simulink model "AUDI"  (R2019b)
settings: Solver=VariableStepAuto  StartTime=0.0  StopTime=100  RelTol=1e-3  AbsTol=1e-3  EnableMultiTasking=on
model workspace (MATLAB code in the model file):
  | v0                 = 15; % Initial vehicle speed
  | wheel_radius = 0.3; % Wheel radius
  | k                   = 1e-2; % Motor losses (W/(N*M)^2)
  | t_torque        = 0.02; % Electric motor time constant
  | gear_ratio     = 4.27;
values from neighbouring files (symbols this model uses):
  dc_battery_internal_resistance = 1e-6    (= 1e-06)    [audi_a3_parameters.m]
  gravitational_acceleration = 9.81    [audi_a3_parameters.m]
  Ki = 60    [audi_a3_parameters.m]
  Kp = 60    [audi_a3_parameters.m]
  speed_controller_lower_limit = -400    [audi_a3_parameters.m]
  speed_controller_upper_limit = 400    [audi_a3_parameters.m]
libraries: fl_lib x36, nesl_utility x11, sdl_lib x5
CloseFcn:
  | try,close(h1_sdl_hybrid_parallel),end
  | clear h1_sdl_hybrid_parallel
  | try,close(h2_sdl_hybrid_parallel),end
  | clear h2_sdl_hybrid_parallel
  | 
  | 
  | clear simlog_sdl_hybrid_parallel
Description:
  | Parallel Hybrid Transmission
settings Model: FPTRunName=Active  Creator=MathWorks  LastModifiedBy=Matheus Elyasha
settings SolverCC: AutoScaleAbsTol=off
settings DataIOCC: LimitDataPoints=on  MaxDataPoints=10000  SaveFormat=Array  SignalLoggingSaveFormat=ModelDataLogs  ReturnWorkspaceOutputs=off  SignalLoggingName=logsout_sdl_hybrid_parallel
settings OptimizationCC: ExpressionDepthLimit=2147483647  LifeSpan=inf
settings DebuggingCC: StateNameClashWarn=warning  PregeneratedLibrarySubsystemCodeDiagnostic=none  SFUnexpectedBacktrackingDiag=warning  SFNoUnconditionalDefaultTransitionDiag=warning  SFExecutionAtInitializationDiag=none  ArithmeticOperatorsInVariantConditions=warning
settings HardwareCC: ProdBitPerPointer=32  ProdBitPerSizeT=32  ProdBitPerPtrDiffT=32  ProdLargestAtomicFloat=None  ProdIntDivRoundTo=Undefined  ProdEndianess=Unspecified  ProdWordSize=32  ProdHWDeviceType=32-bit Generic
settings ModelReferenceCC: PropagateSignalLabelsOutOfModel=off
settings SFSimCC: SimUseLocalCustomCode=off  CustomCodeUndefinedFunction=UseInterfaceOnly
settings RTWCC: RTWUseLocalCustomCode=off
settings CodeAppCC: StateflowObjectComments=on
settings GRTTargetCC: TargetLangStandard=C89/C90 (ANSI)  GeneratePreprocessorConditionals=Disable all  CombineOutputUpdateFcns=off  GRTInterface=on
settings ConfigComp: CovMetricSettings=dw  CovHtmlReporting=on  CovSaveCumulativeToWorkspaceVar=on  CovSaveSingleToWorkspaceVar=on  CovShowResultsExplorer=off  CovExternalEMLEnable=off
settings SimscapeCC: SimscapeLogType=all  SimscapeLogSimulationStatistics=on  SimscapeLogName=simlog_sdl_hybrid_parallel  SimscapeLogDataHistory=10000

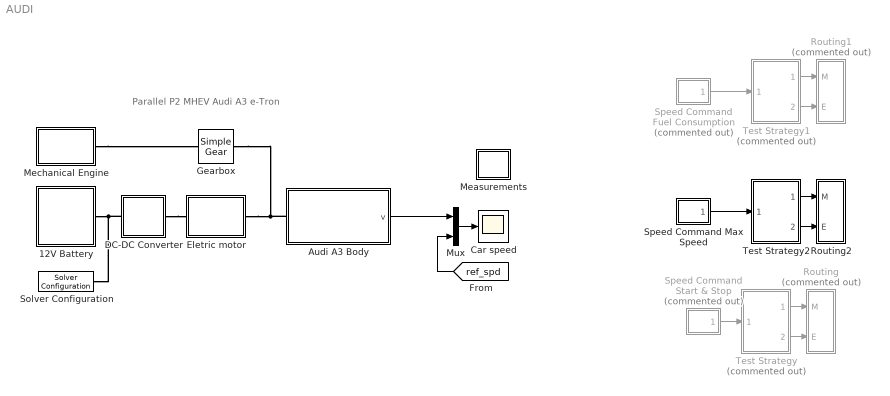
== system AUDI ==
  note: Parallel P2 MHEV Audi A3 e-Tron
  12V Battery : Subsystem
      mask Display:
      | % Plot points to set plot range
      | color('white');plot(1.5, 2.5);plot(-1.5, -2)
      | color('black');
      | % Battery icon
      | plot([0 0], [2.5 1.3])
      | plot([0 0], [-0.6 -1.6])
      | patch([-1 1 1 -1]*0.4, [1 1 -1 -1]*0.15+0.7,[0;0;0]);
      | patch([-1 1 1 -1]*0.4, [1 1 -1 -1]*0.15-0.6,[0;0;0]);
      | patch([-1 1 1 -1]*0.8, [1 1 -1 -1]*0.15+1.3,[0;0;0]);
      | patch([-1 1 1 -1]*0.8, [1 1 -1 -1]*0.15+0.0,[0;0;0]);
  Audi A3 Body : Subsystem
      mask Display:
      | color('white')
      | plot(-120,-60); plot(120,50);
      | color('black')
      | plot(sin(0:0.1:6*pi)*15-70,cos(0:0.1:6*pi)*15-30);
      | plot(sin(0:0.1:6*pi)*15+70,cos(0:0.1:6*pi)*15-30);
      | plot([-88 -95 -99 -99 -95 -75 -65 -50 -46 10 30 34 80 85 90 93 95 93 90 88],[-30 -28 -23 -5 0 5 10 20 21 21 0 -2 -7 -9 -13 -17 -25 -28 -30 -30])
      | plot([-88 -95 -99 -99 -95 -75 -65 -50 -46 10 30 34 80 85 90 93 95 93 90 88],[-30 -28 -23 -5 0 5 10 20 21 21 0 -2 -7 -9 -13 -17 -25 -28 -30 -30]-1)
      | plot([-88 -95 -99 -99 -95 -75 -65 -50 -46 10 30 34 80 85 90 93 95 93 90 88]+1,[-30 -28 -23 -5 0 5 10 20 21 21 0 -2 -7 -9 -13 -17 -25 -28 -30 -30])
      | plot([-50 50],[-30 -30])
  Car speed : Scope
  DC-DC Converter : Subsystem
      mask Display:
      | patch([-0.9 -1 -1 0.9 1 1 -0.9],[-1 -1 -0.9 1 1 0.9 -1],[0 0 0])
      | 
      | patch([-0.8 -0.1 -0.1 -0.8],[0.85 0.85 0.75 0.75],[0 0 0])
      | patch([-0.8 -0.55 -0.55 -0.8],[0.65 0.65 0.55 0.55],[0 0 0])
      | patch([-0.35 -0.1 -0.1 -0.35],[0.65 0.65 0.55 0.55],[0 0 0])
      | 
      | patch([-0.8 -0.1 -0.1 -0.8]*-1,[0.65 0.65 0.55 0.55]*-1,[0 0 0])
      | patch([-0.8 -0.55 -0.55 -0.8]*-1,[0.85 0.85 0.75 0.75]*-1,[0 0 0])
      | patch([-0.35 -0.1 -0.1 -0.35]*-1,[0.85 0.85 0.75 0.75]*-1,[0 0 0])
  Eletric motor : Subsystem
      mask Display:
      | % Circle
      | plot(sin(0:0.1:2.2*pi)*0.9,cos(0:0.1:2.2*pi)*0.9);
      | 
      | % In/out
      | plot([-1.1 -0.9],[0 0]);
      | plot([1.1 0.9],[0 0]);
      | 
      | % 'M'
      | plot([0.5 0.5],[-0.5 0.5]);
      | plot([-0.5 -0.5],[-0.5 0.5]);
      | plot([0.5 0],[0.5 -0.5]);
      | plot([-0.5 0],[0.5 -0.5]);
      | 
      | % Plot points to set plot range
      | color('white');plot(1.9,1.2);plot(-1.9,-1.2)
      | color('black');
  Gearbox : sdl_lib/Gears/Simple Gear  ratio=gear_ratio  rotation_direction=1  friction_model=sdl.enum.gear_efficiencies_load.constant  T_noload=0.1 N*m  T_nom=5 N*m  efficiency_nom=0.8  efficiency=gearbox_efficiency  mu_visc=gearbox_viscous_friction_coefficient_at_B_and_F N*m/(rad/s)  w_thr=0.01 rad/s  pwr_thr=gearbox_follower_power_threshold W  enable_faults=simscape.enum.onoff.off  efficiency_fault=0.05  external_fault=simscape.enum.onoff.off  temporal_fault=simscape.enum.onoff.off  fault_time=5 s  fault_angles=pi / 12 rad  report_fault=1  temperature_TLU=[ 280 300 320 ] K  load_TLU=[ 1 5 10 ] N*m  efficiency_TLU=[ 0.95 0.9 0.85 ]  efficiency_TLU2=[ 0.85 0.8 0.75; 0.95 0.9 0.85; 0.85 0.8 0.7 ]  thermal_mass=50 J/K  T_init=300 K
      settings: SourceProductName=Simscape Driveline
  Measurements : Subsystem
  Mechanical Engine : Subsystem
      mask Display:
      | patch([0 374 374 0 0],[183 40 40 183 183],[1 1 1]);
      | plot([200.294537656123;201.704177092068;202.879954177142;203.81054553527;204.486989062962;204.902770239264;205.053884864158;204.938877621199;204.558856093007;203.917480094638;203.02092642757;201.877829393721;200.499197642409;198.898308151034;197.090578360535;195.093417696999;192.926059909376;191.349221415216], [79.0962651705123;81.4129472419303;83.856642682368;86.4038173688741;89.0299406167901;91.7097214236537;94.4173520353776;97.1267564890293;99.8118417386092;102.446748945347;105.006102512455;107.465254465996;109.80052182835;111.989414698229;114.010852840726;115.845368701499;117.475294889959;118.468271604945])
      | plot([180.070315486255;177.215173525063;174.340173090774;171.473002009205;168.641272705228;165.872256280019;163.192619875453;160.628169854943;158.203603274058;155.942270034374;153.865948011161;151.994633320535;150.346347745932;148.936965178479;147.780058742747;146.886770080143;146.265702048809;145.922835873396;145.861473542603;146.08220600922;146.58290749893;147.358755982674;148.402279615432;149.703428694174;151.249672441989;153.026119686324;155.015662269112;157.199139807684;159.555524219735;162.062122235246;164.694793945081;167.42818528151;170.23597219174;173.091114152932;175.966114587221;178.83328566879;181.665014972767;184.434031397976;185.486929355725], [123.25590763568;123.598773811093;123.660136141886;123.439403675268;122.938702185559;122.162853701815;121.119330069056;119.818180990315;118.2719372425;116.495489998164;114.505947415377;112.322469876805;109.966085464754;107.459487449243;104.826815739408;102.093424402979;99.2856374927491;96.4304955315569;93.5554950972677;90.688324015699;87.8565947117214;85.0875782865128;82.4079418819464;79.8434918614364;77.4189252805513;75.1575920408679;73.081270017655;71.2099553270291;69.5616697524256;68.1522871849724;66.9953807492411;66.1020920866371;65.4810240553025;65.1381578798894;65.0767955490969;65.2975280157144;65.7982295054238;66.5740779891678;66.9481130562871])
      | plot([182.088349247351;182.056804583223;181.962474383197;181.806267098667;181.589687091173;181.314820144583;180.98431337785;180.601349751811;180.169617415534;179.693274187426;179.176907513169;178.625490286111;178.044332955585;177.439032384376;176.815417947876;176.17949539401;175.537389004603;174.895282615196;174.25936006133;173.63574562483;173.030445053621;172.449287723095;171.897870496037;171.38150382178;170.905160593672;170.473428257395;170.090464631356;169.759957864623;169.485090918033;169.268510910539;169.112303626009;169.017973425983;168.986428761855;169.017973425983;169.112303626009;169.268510910539;169.485090918033;169.759957864623;170.090464631356;170.473428257395;170.905160593672;171.38150382178;171.897870496037;172.449287723095;173.030445053621;173.63574562483;174.25936006133;174.895282615196;175.537389004603;176.17949539401;176.815417947876;177.439032384376;178.044332955585;178.625490286111;179.176907513169;179.693274187426;180.169617415534;180.601349751811;180.98431337785;181.314820144583;181.589687091173;181.806267098667;181.962474383197;182.056804583223;182.088349247351;182.088349247351], [94.3432759959251;93.7073437064164;93.0775357924916;92.4599176486499;91.8604372752408;91.2848679959696;90.7387528576339;90.2273512475527;89.7555882427917;89.3280071789786;88.9487258954975;88.6213970784445;88.3491730832641;88.1346755758426;87.9799702844327;87.8865471055612;87.8553057555109;87.8865471055612;87.9799702844327;88.1346755758426;88.3491730832641;88.6213970784445;88.9487258954975;89.3280071789786;89.7555882427917;90.2273512475527;90.7387528576339;91.2848679959696;91.8604372752408;92.4599176486499;93.0775357924916;93.7073437064164;94.3432759959251;94.9792082854337;95.6090161993586;96.2266343432003;96.8261147166093;97.4016839958805;97.9477991342162;98.4592007442974;98.9309637490584;99.3585448128716;99.7378260963527;100.065154913406;100.337378908586;100.551876416008;100.706581707417;100.800004886289;100.831246236339;100.800004886289;100.706581707417;100.551876416008;100.337378908586;100.065154913406;99.7378260963526;99.3585448128716;98.9309637490584;98.4592007442974;97.9477991342162;97.4016839958805;96.8261147166093;96.2266343432003;95.6090161993586;94.9792082854338;94.3432759959251;94.3432759959251])
      | plot([201.615249970928;201.583705306799;201.489375106774;201.333167822243;201.11658781475;200.84172086816;200.511214101427;200.128250475388;199.69651813911;199.220174911002;198.703808236745;198.152391009688;197.571233679162;196.965933107953;196.342318671452;195.706396117586;195.06428972818;194.422183338773;193.786260784907;193.162646348407;192.557345777197;191.976188446671;191.424771219614;190.908404545357;190.432061317249;190.000328980971;189.617365354932;189.286858588199;189.011991641609;188.795411634116;188.639204349585;188.54487414956;188.513329485431;188.54487414956;188.639204349585;188.795411634116;189.011991641609;189.286858588199;189.617365354932;190.000328980971;190.432061317249;190.908404545357;191.424771219614;191.976188446671;192.557345777197;193.162646348407;193.786260784907;194.422183338773;195.06428972818;195.706396117586;196.342318671452;196.965933107953;197.571233679162;198.152391009688;198.703808236745;199.220174911002;199.69651813911;200.128250475388;200.511214101427;200.84172086816;201.11658781475;201.333167822243;201.489375106774;201.583705306799;201.615249970928;201.615249970928], [74.7533852700144;74.1174529805057;73.487645066581;72.8700269227392;72.2705465493302;71.694977270059;71.1488621317233;70.6374605216421;70.165697516881;69.7381164530679;69.3588351695868;69.0315063525339;68.7592823573535;68.5447848499319;68.390079558522;68.2966563796505;68.2654150296003;68.2966563796505;68.390079558522;68.5447848499319;68.7592823573535;69.0315063525339;69.3588351695868;69.7381164530679;70.165697516881;70.6374605216421;71.1488621317233;71.694977270059;72.2705465493302;72.8700269227392;73.487645066581;74.1174529805057;74.7533852700144;75.3893175595231;76.0191254734479;76.6367436172896;77.2362239906986;77.8117932699698;78.3579084083055;78.8693100183867;79.3410730231478;79.7686540869609;80.147935370442;80.4752641874949;80.7474881826754;80.9619856900969;81.1166909815068;81.2101141603783;81.2413555104285;81.2101141603783;81.1166909815068;80.9619856900969;80.7474881826753;80.4752641874949;80.147935370442;79.7686540869609;79.3410730231478;78.8693100183867;78.3579084083055;77.8117932699698;77.2362239906986;76.6367436172896;76.0191254734479;75.3893175595231;74.7533852700145;74.7533852700144])
      | plot([201.615249970928;201.583705306799;201.489375106774;201.333167822243;201.11658781475;200.84172086816;200.511214101427;200.128250475388;199.69651813911;199.220174911002;198.703808236745;198.152391009688;197.571233679162;196.965933107953;196.342318671452;195.706396117586;195.06428972818;194.422183338773;193.786260784907;193.162646348407;192.557345777197;191.976188446671;191.424771219614;190.908404545357;190.432061317249;190.000328980971;189.617365354932;189.286858588199;189.011991641609;188.795411634116;188.639204349585;188.54487414956;188.513329485431;188.54487414956;188.639204349585;188.795411634116;189.011991641609;189.286858588199;189.617365354932;190.000328980971;190.432061317249;190.908404545357;191.424771219614;191.976188446671;192.557345777197;193.162646348407;193.786260784907;194.422183338773;195.06428972818;195.706396117586;196.342318671452;196.965933107953;197.571233679162;198.152391009688;198.703808236745;199.220174911002;199.69651813911;200.128250475388;200.511214101427;200.84172086816;201.11658781475;201.333167822243;201.489375106774;201.583705306799;201.615249970928;201.615249970928], [74.7533852700144;74.1174529805057;73.487645066581;72.8700269227392;72.2705465493302;71.694977270059;71.1488621317233;70.6374605216421;70.165697516881;69.7381164530679;69.3588351695868;69.0315063525339;68.7592823573535;68.5447848499319;68.390079558522;68.2966563796505;68.2654150296003;68.2966563796505;68.390079558522;68.5447848499319;68.7592823573535;69.0315063525339;69.3588351695868;69.7381164530679;70.165697516881;70.6374605216421;71.1488621317233;71.694977270059;72.2705465493302;72.8700269227392;73.487645066581;74.1174529805057;74.7533852700144;75.3893175595231;76.0191254734479;76.6367436172896;77.2362239906986;77.8117932699698;78.3579084083055;78.8693100183867;79.3410730231478;79.7686540869609;80.147935370442;80.4752641874949;80.7474881826754;80.9619856900969;81.1166909815068;81.2101141603783;81.2413555104285;81.2101141603783;81.1166909815068;80.9619856900969;80.7474881826753;80.4752641874949;80.147935370442;79.7686540869609;79.3410730231478;78.8693100183867;78.3579084083055;77.8117932699698;77.2362239906986;76.6367436172896;76.0191254734479;75.3893175595231;74.7533852700145;74.7533852700144])
      | plot([142.90856779553;142.90856779553;208.103220211342;208.103220211342], [139.948037685826;218.181620584801;218.181620584801;139.948037685826])
      | plot([142.90856779553;208.103220211342], [179.064829135314;179.064829135314])
      | plot([149.459528038278;149.459528038278], [179.064829135314;172.576858894899])
      | plot([201.615249970928;201.615249970928], [179.064829135314;172.576858894899])
      | plot([142.90856779553;208.103220211342;208.103220211342;142.90856779553;142.90856779553], [179.064829135314;179.064829135314;152.986968168989;152.986968168989;179.064829135314])
      | plot([142.90856779553;208.103220211342], [192.103759618476;192.103759618476])
      | plot([180.639579193667;200.229469919577], [99.0045361686498;79.4776354450732])
      | plot([173.332738922909;192.92262964882], [87.8553057555109;68.3284050319344])
      | plot([183.663099305704;200.481429928914], [153.553878189996;76.9580353517085])
      | plot([184.544959338382;174.970478983596], [95.0361660216004;153.553878189996])
      | plot([183.474129298702;186.749609420076;206.654450157657;201.615249970928;197.961829835549], [76.9580353517085;62.0923948008567;67.8874750155956;88.1702557671815;87.7923157531768])
      | plot([164.199188584462;187.694459455088], [94.7842060122639;95.1621460262686])
      | plot([175.537389004603;175.285428995267], [106.50034644641;81.9342455361038])
      | plot([142.90856779553;208.103220211342], [172.576858894899;172.576858894899])
      | plot([297.86397353746;317.389525743201], [71.0999651346356;71.0999651346356]+60)
      | plot([269.518472487107;297.86397353746;297.86397353746;269.518472487107;269.518472487107], [85.2727156598121;85.2727156598121;56.927214609459;56.927214609459;85.2727156598121]+60)
      | plot([258.180272066966;269.518472487107;269.518472487107;258.180272066966], [42.7544640842825;42.7544640842825;99.4454661849886;99.4454661849886]+60)
      | plot([108.893966535106;108.245686045801;107.603648851995;106.974038122836;106.362917353826;105.776171972045;105.219452656266;104.698120917834;104.217197466378;103.781313857637;103.394667889039;103.060983172626;102.783473274627;102.564810767061;102.40710148941;102.31186426823;102.280016290024;102.280016290024;102.31186426823;102.40710148941;102.564810767061;102.783473274627;103.060983172626;103.394667889039;103.781313857637;104.217197466378;104.698120917834;105.219452656266;105.776171972045;106.362917353826;106.974038122836;107.603648851995;108.245686045801;108.893966535106;249.67662175186;250.324902241165;250.966939434972;251.596550164131;252.20767093314;252.794416314921;253.3511356307;253.872467369133;254.353390820588;254.78927442933;255.175920397927;255.50960511434;255.787115012339;256.005777519905;256.163486797556;256.258724018736;256.290571996942;256.290571996942;256.258724018736;256.163486797556;256.005777519905;255.787115012339;255.50960511434;255.175920397927;254.78927442933;254.353390820588;253.872467369133;253.3511356307;252.794416314921;252.20767093314;251.596550164131;250.966939434972;250.324902241165;249.67662175186;108.893966535106], [233.173241140321;233.141393162114;233.046155940935;232.888446663284;232.669784155718;232.392274257719;232.058589541306;231.671943572708;231.236059963967;230.755136512511;230.233804774079;229.6770854583;229.090340076519;228.479219307509;227.84960857835;227.207571384544;226.559290895239;46.5338642243296;45.8855837350246;45.2435465412178;44.6139358120588;44.0028150430496;43.4160696612682;42.8593503454891;42.3380186070568;41.8570951556014;41.4212115468599;41.0345655782626;40.7008808618494;40.42337096385;40.2047084562844;40.0469991786335;39.9517619574538;39.9199139792472;39.9199139792472;39.9517619574538;40.0469991786335;40.2047084562844;40.42337096385;40.7008808618494;41.0345655782626;41.4212115468599;41.8570951556014;42.3380186070568;42.8593503454891;43.4160696612682;44.0028150430496;44.6139358120588;45.2435465412178;45.8855837350246;46.5338642243296;226.559290895239;227.207571384544;227.84960857835;228.479219307509;229.090340076519;229.6770854583;230.233804774079;230.755136512511;231.236059963967;231.671943572708;232.058589541306;232.392274257719;232.669784155718;232.888446663284;233.046155940935;233.141393162114;233.173241140321;233.173241140321])
  Mux : Mux  Inputs=2
  Routing : Subsystem  Commented=on
  Routing1 : Subsystem  Commented=on
  Routing2 : Subsystem
  Solver Configuration : nesl_utility/Solver Configuration  PhysicalDomain=network_engine_domain  SubClassName=solver  LeftPortType=input  RightPortType=generic  Tones=[]  Harmonics=[]  SimulateNoise=off  Profile=off  UseLocalSampling=off  EnableSwitchedLinearOptims=on  FrequencyDomain=off  UseCCode=off  RelTol=0.001  AbsTol=1e-06  MinStep=1e-09  ToWorkspace=off  RevertToSquareIcSolve=off  NumHomotopyIterations=100  PhasorMode=off  PhasorModeNumHarmonics=1  DoDC=off  ResidualTolerance=1e-9  UseLocalSolver=off  LocalSolverChoice=NE_PARTITIONING_ADVANCER  LocalSolverSampleTime=0.005  DoFixedCost=off  MaxNonlinIter=5  MaxModeIter=2  LinearAlgebra=auto  EquationFormulation=NE_TIME_EF  DelaysMemoryBudget=1024  AutomaticFiltering=on  FilteringTimeConstant=0.001  PartitionStorageMethod=EXHAUSTIVE  PartitionMemoryBudget=1024  PartitionMethod=ROBUST
  Speed Command Fuel Consumption : Subsystem  Commented=on
  Speed Command Max Speed : Subsystem
  Speed Command Start & Stop : Subsystem  Commented=on
  Test Strategy : Subsystem  Commented=on
  Test Strategy1 : Subsystem  Commented=on
  Test Strategy2 : Subsystem
  wires:
  Audi A3 Body/1(v) -> Mux/1
  Mux/1 -> Car speed/1
  [ref_spd] -> Mux/2
  Test Strategy/1(Motor) -> Routing/1(M)
  Test Strategy/2(Engine) -> Routing/2(E)
  Speed Command Start & Stop/1(Spd) -> Test Strategy/1(Spd)
  Test Strategy1/2(Engine) -> Routing1/2(E)
  Speed Command Fuel Consumption/1(Spd) -> Test Strategy1/1(Spd)
  Test Strategy1/1(Motor) -> Routing1/1(M)
  Speed Command Max Speed/1(Spd) -> Test Strategy2/1(Spd)
  Test Strategy2/2(Engine) -> Routing2/2(E)
  Test Strategy2/1(Motor) -> Routing2/1(M)
  connections:
  Mechanical Engine/RConn1 -- Gearbox/LConn1
  DC-DC Converter/RConn1 -- Eletric motor/RConn1
  Solver Configuration/RConn1 -- 12V Battery/LConn1 -- DC-DC Converter/LConn1
  Gearbox/RConn1 -- Eletric motor/LConn1 -- Audi A3 Body/LConn1

== system AUDI/12V Battery ==
  Calculations : Subsystem
  Current Sensor : fl_lib/Electrical/Electrical Sensors/Current Sensor
  DC Voltage Source : fl_lib/Electrical/Electrical Sources/DC Voltage Source  v0=dc_voltage_battery V
  ERef : fl_lib/Electrical/Electrical Elements/Electrical Reference
  Internal Resistance : fl_lib/Electrical/Electrical Elements/Resistor  R=dc_battery_internal_resistance Ohm  i_specify=off  i_priority=High  i=0 A  i_nominal_specify=off  i_nominal_unit=A  i_nominal_value=1  v_specify=off  v_priority=High  v=0 V  v_nominal_specify=off  v_nominal_unit=V  v_nominal_value=1
  Voltage Sensor : fl_lib/Electrical/Electrical Sensors/Voltage Sensor
  V : PMIOPort  Side=Left
  connections:
  Voltage Sensor/RConn2 -- Current Sensor/LConn1 -- ERef/LConn1
  Current Sensor/RConn1 -- Calculations/LConn2
  Voltage Sensor/RConn1 -- Calculations/LConn1
  Current Sensor/RConn2 -- DC Voltage Source/RConn1
  Voltage Sensor/LConn1 -- V/RConn1 -- Internal Resistance/RConn1
  DC Voltage Source/LConn1 -- Internal Resistance/LConn1

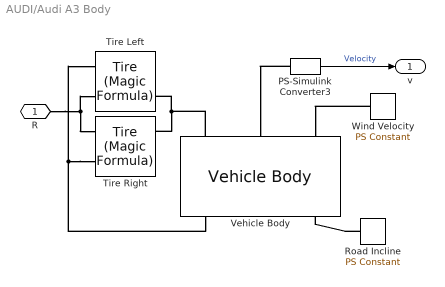
== system AUDI/Audi A3 Body ==
  PS-Simulink Converter3 : nesl_utility/PS-Simulink Converter  PhysicalDomain=network_engine_domain  SubClassName=ps_output  LeftPortType=input  RightPortType=output  PseudoPeriodic=off  Frequencies=[]  Unit=km/hr  AffineConversion=off
  Road Incline : fl_lib/Physical Signals/Sources/PS Constant  constant=0
  Tire Left : sdl_lib/Tires & Vehicles/Tire (Magic Formula)  parameterization=sdl.enum.magic_tire_model.peak  F_z1=left_rated_vertical_load N  F_x1=left_peak_longitudinal_force_at_rated_load N  kappa1=left_peak_force  B_m=10  C_m=1.9  D_m=1  E_m=0.97  fz0=4e+3 N  p_Cx=1.685  p_Dx=[ 1.21 -0.037 ]  p_Ex=[ 0.344 0.095 -0.02 0 ]  p_Kx=[ 21.51 -0.163 0.245 ]  p_Hx=[ -0.002 0.002 ]  p_Vx=[ 0 0 ]  v_tr_thr=left_velocity_threshold m/s  r_e=wheel_radius m  model_compliance=0  stiffness=1e+6 N/m  damping=1000 N/(m/s)  model_inertia=1  inertia=left_tire_inertia kg*m^2  initial_velocity=v0/wheel_radius rad/s  model_resistance=0  resistance_model=1  coeff=0.015  p_tire=2.5e+5 Pa  alpha=-0.003  beta=0.97  coeff_a=0.008399999999999999  coeff_b=6.2e-4 s/m  coeff_c=1.6e-4 s^2/m^2  v_thr=0.001 m/s
      settings: SourceProductName=Simscape Driveline
  Tire Right : sdl_lib/Tires & Vehicles/Tire (Magic Formula)  parameterization=sdl.enum.magic_tire_model.peak  F_z1=right_rated_vertical_load N  F_x1=right_peak_longitudinal_force_at_rated_load N  kappa1=right_peak_force  B_m=10  C_m=1.9  D_m=1  E_m=0.97  fz0=4e+3 N  p_Cx=1.685  p_Dx=[ 1.21 -0.037 ]  p_Ex=[ 0.344 0.095 -0.02 0 ]  p_Kx=[ 21.51 -0.163 0.245 ]  p_Hx=[ -0.002 0.002 ]  p_Vx=[ 0 0 ]  v_tr_thr=right_velocity_threshold m/s  r_e=wheel_radius m  model_compliance=0  stiffness=1e+6 N/m  damping=1000 N/(m/s)  model_inertia=1  inertia=right_tire_inertia kg*m^2  initial_velocity=v0/wheel_radius rad/s  model_resistance=0  resistance_model=1  coeff=0.015  p_tire=2.5e+5 Pa  alpha=-0.003  beta=0.97  coeff_a=0.008399999999999999  coeff_b=6.2e-4 s/m  coeff_c=1.6e-4 s^2/m^2  v_thr=0.001 m/s
      settings: SourceProductName=Simscape Driveline
  Vehicle Body : sdl_lib/Tires & Vehicles/Vehicle Body  mass=audi_mass kg  n_w=number_wheels_per_axle  x_f=horizontal_distance_from_CG_to_front_axle m  x_r=horizontal_distance_from_CG_to_rear_axle m  y_c=CG_height_above_ground m  mass_var=simscape.enum.onoff.off  model_pitch=simscape.enum.onoff.off  inertia=4000 kg*m^2  suspension_model=sdl.enum.linearTLU.linear  k_f=1e4 N/m  b_f=1e4 N/(m/s)  k_r=1e4 N/m  b_r=1e4 N/(m/s)  k_f_TLU=[-2000, -1000, 0, 1000, 2000] N  x_f_TLU=[-.4, -.2, 0, .2, .4] m  b_f_TLU=[-200, -100, 0, 100, 200] N  v_f_TLU=[-4, -2, 0, 2, 4] m/s  k_r_TLU=[-2000, -1000, 0, 1000, 2000] N  x_r_TLU=[-.4, -.2, 0, .2, .4] m  b_r_TLU=[-200, -100, 0, 100, 200] N  v_r_TLU=[-4, -2, 0, 2, 4] m/s  interp_method=simscape.enum.interpolation.linear  extrap_method=simscape.enum.extrapolation.linear  model_hardstop=simscape.enum.onoff.off  upper_bound_f=.25 m  lower_bound_f=-.25 m  stop_k_f=1e6 N/m  stop_b_f=150 N/(m/s)  upper_bound_r=.25 m  lower_bound_r=-.25 m  stop_k_r=1e6 N/m  stop_b_r=150 N/(m/s)  initial_pitch=0 rad  initial_pitch_rate=0 rad/s  g=gravitational_acceleration m/s^2  liftoff_warning=simscape.enum.onoff.off  area=front_area m^2  Cd=drag_coefficient  rho=air_density kg/m^3  v_specify=on  v_priority=High  v=v0 m/s  v_nominal_specify=off  v_nominal_unit=m/s  v_nominal_value=1
      settings: SourceProductName=Simscape Driveline
  Wind Velocity : fl_lib/Physical Signals/Sources/PS Constant  constant=0
  R : PMIOPort  Side=Left
  v : Outport  VectorParamsAs1DForOutWhenUnconnected=off
  wires:
  PS-Simulink Converter3/1 -> v/1  "Velocity"
  connections:
  Tire Right/LConn1 -- Tire Left/LConn1 -- Vehicle Body/RConn1
  R/RConn1 -- Tire Left/LConn2 -- Tire Right/LConn2
  Vehicle Body/LConn1 -- Tire Left/RConn2 -- Tire Right/RConn2
  PS-Simulink Converter3/LConn1 -- Vehicle Body/LConn2
  Road Incline/RConn1 -- Vehicle Body/RConn3
  Wind Velocity/RConn1 -- Vehicle Body/LConn3

== system AUDI/DC-DC Converter ==
  ERef High : fl_lib/Electrical/Electrical Elements/Electrical Reference
  ERef Low : fl_lib/Electrical/Electrical Elements/Electrical Reference
  Ideal DC-DC Voltage Converter : fl_lib/Electrical/Electrical Elements/Ideal Transformer  n=dc_dc_converter_winding_ration  i1_specify=off  i1_priority=None  i1=0 A  i1_nominal_specify=off  i1_nominal_unit=A  i1_nominal_value=1  v1_specify=off  v1_priority=None  v1=0 V  v1_nominal_specify=off  v1_nominal_unit=V  v1_nominal_value=1  i2_specify=off  i2_priority=None  i2=0 A  i2_nominal_specify=off  i2_nominal_unit=A  i2_nominal_value=1  v2_specify=off  v2_priority=None  v2=0 V  v2_nominal_specify=off  v2_nominal_unit=V  v2_nominal_value=1
      settings: SourceProductName=Simscape  SourceProductBaseCode=SS
  L : PMIOPort  Tag=PMCPort  Side=Left
  H : PMIOPort  Port=2  Side=Right
  connections:
  Ideal DC-DC Voltage Converter/LConn1 -- L/RConn1
  Ideal DC-DC Voltage Converter/LConn2 -- ERef Low/LConn1
  H/RConn1 -- Ideal DC-DC Voltage Converter/RConn1
  ERef High/LConn1 -- Ideal DC-DC Voltage Converter/RConn2

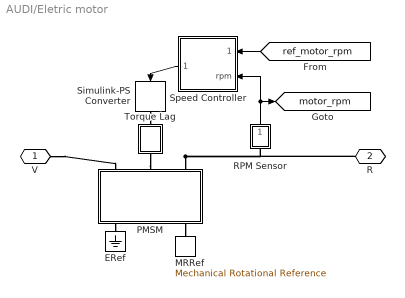
== system AUDI/Eletric motor ==
  ERef : fl_lib/Electrical/Electrical Elements/Electrical Reference
  MRRef : fl_lib/Mechanical/Rotational Elements/Mechanical Rotational Reference
  PMSM : Subsystem
  RPM Sensor : Subsystem
      mask Display: disp('S')
  Simulink-PS Converter : nesl_utility/Simulink-PS Converter  PhysicalDomain=network_engine_domain  SubClassName=ps_input  LeftPortType=input  RightPortType=output  PseudoPeriodic=off  Frequencies=[]  NoiseDistribution=none  NoiseParameters=[]  Unit=N*m  AffineConversion=off  FilteringAndDerivatives=zero  SimscapeFilterOrder=1  InputFilterTimeConstant=.001  UdotUserProvided=0
  Speed Controller : Subsystem
  Torque Lag : Subsystem
  V : PMIOPort  Side=Right
  R : PMIOPort  Port=2  Side=Left
  tag scope: motor_rpm=global
  wires:
  RPM Sensor/1(rpm) -> Speed Controller/2(rpm), [motor_rpm]
  [ref_motor_rpm] -> Speed Controller/1(rpm_ref)
  Speed Controller/1(T_ref) -> Simulink-PS Converter/1
  connections:
  Simulink-PS Converter/RConn1 -- Torque Lag/LConn1
  PMSM/RConn3 -- MRRef/LConn1
  PMSM/RConn1 -- ERef/LConn1
  V/RConn1 -- PMSM/LConn1
  Torque Lag/RConn1 -- PMSM/LConn2
  PMSM/LConn3 -- R/RConn1 -- RPM Sensor/LConn1

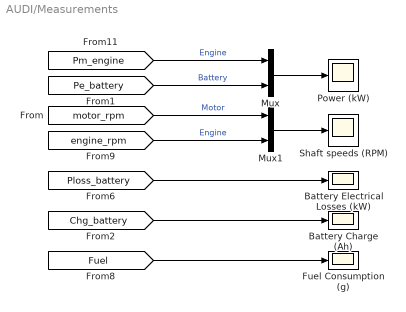
== system AUDI/Measurements ==
  Battery Charge (Ah) : Scope
  Battery Electrical Losses (kW) : Scope
  Fuel Consumption (g) : Scope
  Mux : Mux  Inputs=2
  Mux1 : Mux  Inputs=2
  Power (kW) : Scope
  Shaft speeds (RPM) : Scope
  wires:
  Mux/1 -> Power (kW)/1
  Mux1/1 -> Shaft speeds (RPM)/1
  [motor_rpm] -> Mux1/1  "Motor"
  [engine_rpm] -> Mux1/2  "Engine"
  [Pm_engine] -> Mux/1  "Engine"
  [Pe_battery] -> Mux/2  "Battery"
  [Ploss_battery] -> Battery Electrical Losses (kW)/1
  [Fuel] -> Fuel Consumption (g)/1
  [Chg_battery] -> Battery Charge (Ah)/1

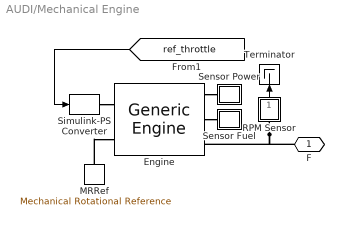
== system AUDI/Mechanical Engine ==
  Engine : sdl_lib/Engines/Generic Engine  model_parameterization=1  engine_type=1  P_max=engine_max_power W  w_P_max=engine_speed_at_max_power rpm  w_max=engine_max_speed rpm  w_min=engine_stall_speed rpm  w_tab=[ 500 1000 2e+3 3e+3 4e+3 5e+3 6e+3 7e+3 ] rpm  trq_tab=[ 380 380 380 380 350 280 200 80 ] N*m  pwr_tab=[ 2e+4 4e+4 7.8e+4 1.2e+5 1.45e+5 1.48e+5 1.25e+5 6e+4 ] W  interp_method=simscape.enum.interpolation.linear  model_inertia=1  inertia=engine_inertia kg*m^2  initial_velocity=v0/wheel_radius*gear_ratio rad/s  model_time_constant=1  time_constant=engine_time_constant s  T0=engine_initial_normalized_throttle  w_thr=engine_speed_threshold rpm  idle_speed=0  idle_speed_reference=1000 rpm  tau_controller=1 s  idle_w_thr=1 rpm  redline=0  redline_speed=5000 rpm  tau_redline=1 s  redline_w_thr=1 rpm  fc_model=4  fc_per_rev=25 mg/rev  displaced_volume=engine_displaced_volume cm^3  rev_per_cycle=engine_revolutions_per_cycle  fc_w_tab=engine_speed_vector rpm  fc_trq_tab=[ 0 80 160 200 240 320 360 400 ] N*m  fc_tab=[ 0.5 0.9 1.4 1.6 1.9 2.7 3.4 4.4; 1 1.7 2.7 3.1 3.6 5 6 7.4; 1.4 2.7 4 4.8 5.6 7.5 8.5 10.5; 2 3.6 5.8 6.7 8 10.4 11.7 13.3; 2.5 4.8 7.9 9.4 10.8 14 16.2 18.6; 3.1 6 10.3 11.9 13.8 18.4 22 26.5 ] g/s  bmep_tab=engine_brake_mean_effective_pressure_vector kPa  bsfc_tab=engine_brake_specific_fuel_consumption_table g/hr/kW  fc_interp_method=simscape.enum.interpolation.linear
      settings: SourceProductName=Simscape Driveline  SourceProductBaseCode=LD  InternalSimscapePortConfiguration="{\"Bottom\":[],\"Left\":[{\"id\":\"T\",\"label\":\"T\",\"type\":\"input\"},{\"id\":\"B\",\"label\":\"B\",\"type\":\"foundation.mechanical.rotational.rotational\"}],\"Right\":[{\"id\":\"P\",\"label\":\"P\",\"type\":\"output\"},{\"id\":\"FC\",\"label\":\"FC\",\"type\":\"output\"},{\"id\":\"F\",\"label\":\"F\",\"type\":\"foundation.mechanical.rotational.rotational\"}],\"Top\":[]}"
  MRRef : fl_lib/Mechanical/Rotational Elements/Mechanical Rotational Reference
  RPM Sensor : Subsystem
      mask Display: disp('S');
  Sensor Fuel : Subsystem
  Sensor Power : Subsystem
  Simulink-PS Converter : nesl_utility/Simulink-PS Converter  PhysicalDomain=network_engine_domain  SubClassName=ps_input  LeftPortType=input  RightPortType=output  PseudoPeriodic=off  Frequencies=[]  NoiseDistribution=none  NoiseParameters=[]  Unit=1  AffineConversion=off  FilteringAndDerivatives=zero  SimscapeFilterOrder=1  InputFilterTimeConstant=.001  UdotUserProvided=0
  Terminator : Terminator
  F : PMIOPort  Side=Right
  wires:
  [ref_throttle] -> Simulink-PS Converter/1
  RPM Sensor/1(rpm) -> Terminator/1
  connections:
  Engine/RConn2 -- Sensor Fuel/LConn1
  Engine/RConn1 -- Sensor Power/LConn1
  Simulink-PS Converter/RConn1 -- Engine/LConn1
  MRRef/LConn1 -- Engine/LConn2
  RPM Sensor/LConn1 -- Engine/RConn3 -- F/RConn1

== system AUDI/Routing ==
  M : Inport
  E : Inport  Port=2
  tag scope: ref_motor_rpm=global, ref_throttle=global
  wires:
  M/1 -> [ref_motor_rpm]
  E/1 -> [ref_throttle]

== system AUDI/Routing1 ==
  M : Inport
  E : Inport  Port=2
  tag scope: ref_motor_rpm=global, ref_throttle=global
  wires:
  M/1 -> [ref_motor_rpm]
  E/1 -> [ref_throttle]

== system AUDI/Routing2 ==
  M : Inport
  E : Inport  Port=2
  tag scope: ref_motor_rpm=global, ref_throttle=global
  wires:
  M/1 -> [ref_motor_rpm]
  E/1 -> [ref_throttle]

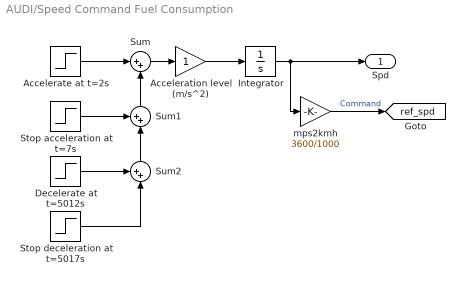
== system AUDI/Speed Command Fuel Consumption ==
  Accelerate at t=2s : Step  Time=2  SampleTime=0
  Acceleration level (m/s^2) : Gain
  Decelerate at t=5012s : Step  Time=12+5000  After=-1  SampleTime=0
  Integrator : Integrator  InitialCondition=v0
  Stop acceleration at t=7s : Step  Time=7  After=-1  SampleTime=0
  Stop deceleration at t=5017s : Step  Time=17+5000  SampleTime=0
  Sum : Sum  Inputs=|++
  Sum1 : Sum  Inputs=++|
  Sum2 : Sum  Inputs=++|
  mps2kmh : Gain  Gain=3600/1000
  Spd : Outport  VectorParamsAs1DForOutWhenUnconnected=off
  tag scope: ref_spd=global
  wires:
  mps2kmh/1 -> [ref_spd]  "Command"
  Stop deceleration at t=5017s/1 -> Sum2/2
  Decelerate at t=5012s/1 -> Sum2/1
  Acceleration level (m/s^2)/1 -> Integrator/1
  Sum2/1 -> Sum1/2
  Sum1/1 -> Sum/2
  Stop acceleration at t=7s/1 -> Sum1/1
  Integrator/1 -> Spd/1, mps2kmh/1
  Sum/1 -> Acceleration level (m/s^2)/1
  Accelerate at t=2s/1 -> Sum/1

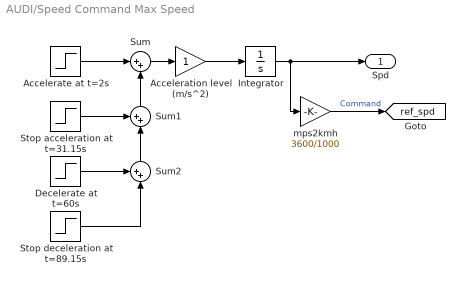
== system AUDI/Speed Command Max Speed ==
  Accelerate at t=2s : Step  Time=2  SampleTime=0
  Acceleration level (m/s^2) : Gain
  Decelerate at t=60s : Step  Time=60  After=-1  SampleTime=0
  Integrator : Integrator  InitialCondition=v0
  "Stop acceleration at t=31.15s " : Step  Time=31.15  After=-1  SampleTime=0
  Stop deceleration at t=89.15s : Step  Time=60+29.15  SampleTime=0
  Sum : Sum  Inputs=|++
  Sum1 : Sum  Inputs=++|
  Sum2 : Sum  Inputs=++|
  mps2kmh : Gain  Gain=3600/1000
  Spd : Outport  VectorParamsAs1DForOutWhenUnconnected=off
  tag scope: ref_spd=global
  wires:
  mps2kmh/1 -> [ref_spd]  "Command"
  Stop deceleration at t=89.15s/1 -> Sum2/2
  Decelerate at t=60s/1 -> Sum2/1
  Acceleration level (m/s^2)/1 -> Integrator/1
  Sum2/1 -> Sum1/2
  Sum1/1 -> Sum/2
  "Stop acceleration at t=31.15s "/1 -> Sum1/1
  Integrator/1 -> Spd/1, mps2kmh/1
  Sum/1 -> Acceleration level (m/s^2)/1
  Accelerate at t=2s/1 -> Sum/1

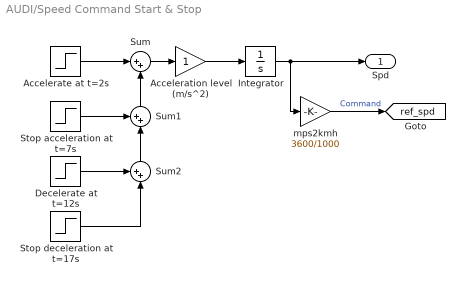
== system AUDI/Speed Command Start & Stop ==
  Accelerate at t=2s : Step  Time=2  SampleTime=0
  Acceleration level (m/s^2) : Gain
  Decelerate at t=12s : Step  Time=12  After=-1  SampleTime=0
  Integrator : Integrator  InitialCondition=v0
  Stop acceleration at t=7s : Step  Time=7  After=-1  SampleTime=0
  Stop deceleration at t=17s : Step  Time=17  SampleTime=0
  Sum : Sum  Inputs=|++
  Sum1 : Sum  Inputs=++|
  Sum2 : Sum  Inputs=++|
  mps2kmh : Gain  Gain=3600/1000
  Spd : Outport  VectorParamsAs1DForOutWhenUnconnected=off
  tag scope: ref_spd=global
  wires:
  mps2kmh/1 -> [ref_spd]  "Command"
  Stop deceleration at t=17s/1 -> Sum2/2
  Decelerate at t=12s/1 -> Sum2/1
  Acceleration level (m/s^2)/1 -> Integrator/1
  Sum2/1 -> Sum1/2
  Sum1/1 -> Sum/2
  Stop acceleration at t=7s/1 -> Sum1/1
  Integrator/1 -> Spd/1, mps2kmh/1
  Sum/1 -> Acceleration level (m/s^2)/1
  Accelerate at t=2s/1 -> Sum/1

== system AUDI/Test Strategy ==
  note: Engine throttle demand has been set so that at the starting condition
      | the combustion engine is providing just enough power to keep the vehicle
      | moving at constant speed, and hence battery power is close to zero. The
      | motor RPM demand is set to track the demanded vehicle speed.
  Spd : Inport
  Convert to wheel RPM : Gain  Gain=60/(2*pi)/wheel_radius
  Engine throttle demand : Constant  Value=0.11
  Motor : Outport  VectorParamsAs1DForOutWhenUnconnected=off
  Engine : Outport  Port=2  VectorParamsAs1DForOutWhenUnconnected=off
  wires:
  Spd/1 -> Convert to wheel RPM/1
  Convert to wheel RPM/1 -> Motor/1
  Engine throttle demand/1 -> Engine/1

== system AUDI/Test Strategy1 ==
  note: Engine throttle demand has been set so that at the starting condition
      | the combustion engine is providing just enough power to keep the vehicle
      | moving at constant speed, and hence battery power is close to zero. The
      | motor RPM demand is set to track the demanded vehicle speed.
  Spd : Inport
  Convert to wheel RPM : Gain  Gain=60/(2*pi)/wheel_radius
  Engine throttle demand : Constant  Value=0.11
  Motor : Outport  VectorParamsAs1DForOutWhenUnconnected=off
  Engine : Outport  Port=2  VectorParamsAs1DForOutWhenUnconnected=off
  wires:
  Spd/1 -> Convert to wheel RPM/1
  Convert to wheel RPM/1 -> Motor/1
  Engine throttle demand/1 -> Engine/1

== system AUDI/Test Strategy2 ==
  note: Engine throttle demand has been set so that at the starting condition
      | the combustion engine is providing just enough power to keep the vehicle
      | moving at constant speed, and hence battery power is close to zero. The
      | motor RPM demand is set to track the demanded vehicle speed.
  Spd : Inport
  Convert to wheel RPM : Gain  Gain=60/(2*pi)/wheel_radius
  Engine throttle demand : Constant  Value=0.11
  Motor : Outport  VectorParamsAs1DForOutWhenUnconnected=off
  Engine : Outport  Port=2  VectorParamsAs1DForOutWhenUnconnected=off
  wires:
  Spd/1 -> Convert to wheel RPM/1
  Convert to wheel RPM/1 -> Motor/1
  Engine throttle demand/1 -> Engine/1

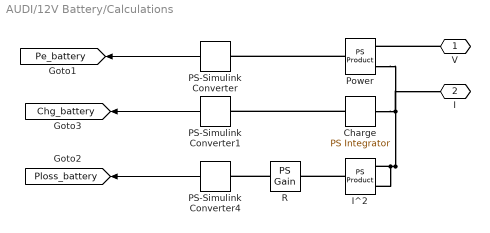
== system AUDI/12V Battery/Calculations ==
  Charge : fl_lib/Physical Signals/Linear Operators/PS Integrator  x0=150 A*hr
      settings: SourceProductName=Simscape  SourceProductBaseCode=SS
  I^2 : fl_lib/Physical Signals/Functions/PS Product
      settings: SourceProductName=Simscape
  PS-Simulink Converter : nesl_utility/PS-Simulink Converter  PhysicalDomain=network_engine_domain  SubClassName=ps_output  LeftPortType=input  RightPortType=output  PseudoPeriodic=off  Frequencies=[]  Unit=kW  AffineConversion=off
  PS-Simulink Converter1 : nesl_utility/PS-Simulink Converter  PhysicalDomain=network_engine_domain  SubClassName=ps_output  LeftPortType=input  RightPortType=output  PseudoPeriodic=off  Frequencies=[]  Unit=A*hr  AffineConversion=off
  PS-Simulink Converter4 : nesl_utility/PS-Simulink Converter  PhysicalDomain=network_engine_domain  SubClassName=ps_output  LeftPortType=input  RightPortType=output  PseudoPeriodic=off  Frequencies=[]  Unit=kW  AffineConversion=off
  Power : fl_lib/Physical Signals/Functions/PS Product
      settings: SourceProductName=Simscape
  R : fl_lib/Physical Signals/Functions/PS Gain  gain=0.05 V/A
  V : PMIOPort  Side=Left
  I : PMIOPort  Port=2  Side=Left
  tag scope: Chg_battery=global, Pe_battery=global, Ploss_battery=global
  wires:
  PS-Simulink Converter/1 -> [Pe_battery]
  PS-Simulink Converter1/1 -> [Chg_battery]
  PS-Simulink Converter4/1 -> [Ploss_battery]
  connections:
  Charge/RConn1 -- PS-Simulink Converter1/LConn1
  Power/RConn1 -- PS-Simulink Converter/LConn1
  V/RConn1 -- Power/LConn1
  I^2/LConn1 -- Charge/LConn1 -- Power/LConn2 -- I/RConn1 -- I^2/LConn2
  I^2/RConn1 -- R/LConn1
  R/RConn1 -- PS-Simulink Converter4/LConn1

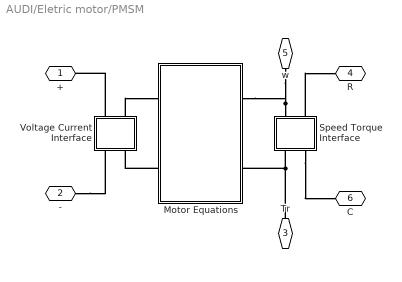
== system AUDI/Eletric motor/PMSM ==
  Motor Equations : Subsystem
  Speed Torque Interface : Subsystem
  Voltage Current Interface : Subsystem
  + : PMIOPort  Side=Left
  - : PMIOPort  Port=2  Side=Right
  Tr : PMIOPort  Port=3  Side=Left
  R : PMIOPort  Port=4  Side=Left
  w : PMIOPort  Port=5  Side=Right
  C : PMIOPort  Port=6  Side=Right
  connections:
  Motor Equations/LConn2 -- Voltage Current Interface/RConn2
  Speed Torque Interface/LConn1 -- Motor Equations/RConn1 -- w/RConn1
  Voltage Current Interface/LConn2 -- Motor Equations/LConn1
  Tr/RConn1 -- Speed Torque Interface/RConn1 -- Motor Equations/RConn2
  Speed Torque Interface/RConn2 -- C/RConn1
  Speed Torque Interface/LConn2 -- R/RConn1
  -/RConn1 -- Voltage Current Interface/RConn1
  Voltage Current Interface/LConn1 -- +/RConn1

== system AUDI/Eletric motor/RPM Sensor ==
  Mechanical Rotational Reference : fl_lib/Mechanical/Rotational Elements/Mechanical Rotational Reference
  Motion Sensor : fl_lib/Mechanical/Mechanical Sensors/Ideal Rotational Motion Sensor  offset=electric_motor_motion_sensor rad
  PS-Simulink Converter 2 : nesl_utility/PS-Simulink Converter  PhysicalDomain=network_engine_domain  SubClassName=ps_output  LeftPortType=input  RightPortType=output  PseudoPeriodic=off  Frequencies=[]  Unit=rpm  AffineConversion=off
  R : PMIOPort  Side=Left
  rpm : Outport  VectorParamsAs1DForOutWhenUnconnected=off
  wires:
  PS-Simulink Converter 2/1 -> rpm/1
  connections:
  R/RConn1 -- Motion Sensor/LConn1
  Motion Sensor/RConn1 -- Mechanical Rotational Reference/LConn1
  Motion Sensor/RConn2 -- PS-Simulink Converter 2/LConn1

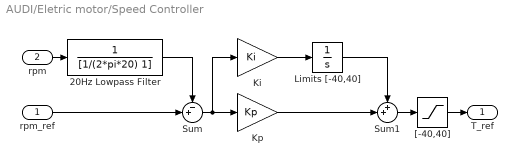
== system AUDI/Eletric motor/Speed Controller ==
  rpm_ref : Inport
  rpm : Inport  Port=2
  20Hz Lowpass Filter : TransferFcn  Denominator=[1/(2*pi*20) 1]
  Ki : Gain  Gain=Ki
  Kp : Gain  Gain=Kp
  Limits [-40,40] : Integrator  LimitOutput=on  UpperSaturationLimit=40  LowerSaturationLimit=-40
  Sum : Sum  Inputs=-+|
  Sum1 : Sum  Inputs=++|
  "[-40,40]" : Saturate  UpperLimit=speed_controller_upper_limit  LowerLimit=speed_controller_lower_limit
  T_ref : Outport  VectorParamsAs1DForOutWhenUnconnected=off
  wires:
  "[-40,40]"/1 -> T_ref/1
  20Hz Lowpass Filter/1 -> Sum/1
  Limits [-40,40]/1 -> Sum1/1
  Kp/1 -> Sum1/2
  Ki/1 -> Limits [-40,40]/1
  Sum/1 -> Kp/1, Ki/1
  Sum1/1 -> "[-40,40]"/1
  rpm/1 -> 20Hz Lowpass Filter/1
  rpm_ref/1 -> Sum/2

== system AUDI/Eletric motor/Torque Lag ==
  0.2 second lag : fl_lib/Physical Signals/Functions/PS Gain  gain=1/t_torque 1/s
  PS Integrator : fl_lib/Physical Signals/Linear Operators/PS Integrator  x0=0 N*m
      settings: SourceProductName=Simscape  SourceProductBaseCode=SS
  PS Subtract : fl_lib/Physical Signals/Functions/PS Subtract
      settings: SourceProductName=Simscape
  i : PMIOPort  Side=Left
  o : PMIOPort  Port=2  Side=Right
  connections:
  PS Subtract/RConn1 -- 0.2 second lag/LConn1
  0.2 second lag/RConn1 -- PS Integrator/LConn1
  PS Integrator/RConn1 -- o/RConn1 -- PS Subtract/LConn2
  i/RConn1 -- PS Subtract/LConn1

== system AUDI/Mechanical Engine/RPM Sensor ==
  MRR : fl_lib/Mechanical/Rotational Elements/Mechanical Rotational Reference
  Motion Sensor : fl_lib/Mechanical/Mechanical Sensors/Ideal Rotational Motion Sensor  offset=motion_sensor_initial_angle rad
  PS2S : nesl_utility/PS-Simulink Converter  PhysicalDomain=network_engine_domain  SubClassName=ps_output  LeftPortType=input  RightPortType=output  PseudoPeriodic=off  Frequencies=[]  Unit=rpm  AffineConversion=off
  Sensor Dynamics : TransferFcn  Denominator=[0.01 1]
  F : PMIOPort  Side=Left
  rpm : Outport  VectorParamsAs1DForOutWhenUnconnected=off
  tag scope: engine_rpm=global
  wires:
  Sensor Dynamics/1 -> rpm/1
  PS2S/1 -> [engine_rpm], Sensor Dynamics/1
  connections:
  MRR/LConn1 -- Motion Sensor/RConn1
  Motion Sensor/RConn2 -- PS2S/LConn1
  F/RConn1 -- Motion Sensor/LConn1

== system AUDI/Mechanical Engine/Sensor Fuel ==
  Integrator : Integrator
  PS2S2 : nesl_utility/PS-Simulink Converter  PhysicalDomain=network_engine_domain  SubClassName=ps_output  LeftPortType=input  RightPortType=output  PseudoPeriodic=off  Frequencies=[]  Unit=g/s  AffineConversion=off
  FC : PMIOPort  Side=Left
  tag scope: Fuel=global
  wires:
  Integrator/1 -> [Fuel]
  PS2S2/1 -> Integrator/1
  connections:
  FC/RConn1 -- PS2S2/LConn1

== system AUDI/Mechanical Engine/Sensor Power ==
  PS2S1 : nesl_utility/PS-Simulink Converter  PhysicalDomain=network_engine_domain  SubClassName=ps_output  LeftPortType=input  RightPortType=output  PseudoPeriodic=off  Frequencies=[]  Unit=kW  AffineConversion=off
  P : PMIOPort  Side=Left
  tag scope: Pm_engine=global
  wires:
  PS2S1/1 -> [Pm_engine]
  connections:
  P/RConn1 -- PS2S1/LConn1

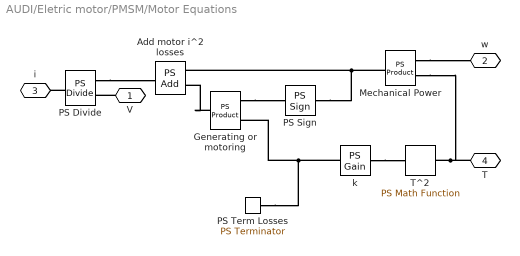
== system AUDI/Eletric motor/PMSM/Motor Equations ==
  Add motor i^2 losses : fl_lib/Physical Signals/Functions/PS Add
  Generating or motoring : fl_lib/Physical Signals/Functions/PS Product
      settings: SourceProductName=Simscape
  Mechanical Power : fl_lib/Physical Signals/Functions/PS Product
      settings: SourceProductName=Simscape
  PS Divide : fl_lib/Physical Signals/Functions/PS Divide
      settings: SourceProductName=Simscape  SourceProductBaseCode=SS
  PS Sign : fl_lib/Physical Signals/Nonlinear Operators/PS Sign
      settings: SourceProductName=Simscape  SourceProductBaseCode=SS  InternalSimscapePortConfiguration="{\"Bottom\":[],\"Left\":[{\"id\":\"I\",\"label\":\"\",\"type\":\"input\"}],\"Right\":[{\"id\":\"O\",\"label\":\"\",\"type\":\"output\"}],\"Top\":[]}"
  PS Term Losses : fl_lib/Physical Signals/Sinks/PS Terminator
      settings: SourceProductName=Simscape
  T^2 : fl_lib/Physical Signals/Functions/PS Math Function  fcn_choice=7
      settings: SourceProductName=Simscape  SourceProductBaseCode=SS
  k : fl_lib/Physical Signals/Functions/PS Gain  gain=k 1/(N*m*s)
  V : PMIOPort  Side=Left
  w : PMIOPort  Port=2  Side=Right
  i : PMIOPort  Port=3  Side=Left
  T : PMIOPort  Port=4  Side=Right
  connections:
  V/RConn1 -- PS Divide/LConn2
  PS Divide/RConn1 -- i/RConn1
  Mechanical Power/RConn1 -- Add motor i^2 losses/LConn1 -- PS Sign/LConn1
  Generating or motoring/RConn1 -- Add motor i^2 losses/LConn2
  PS Divide/LConn1 -- Add motor i^2 losses/RConn1
  Mechanical Power/LConn1 -- w/RConn1
  PS Term Losses/LConn1 -- k/RConn1 -- Generating or motoring/LConn2
  T^2/LConn1 -- T/RConn1 -- Mechanical Power/LConn2
  k/LConn1 -- T^2/RConn1
  Generating or motoring/LConn1 -- PS Sign/RConn1

== system AUDI/Eletric motor/PMSM/Speed Torque Interface ==
  Motion Sensor : fl_lib/Mechanical/Mechanical Sensors/Ideal Rotational Motion Sensor  offset=0 rad
  Torque Source : fl_lib/Mechanical/Mechanical Sources/Ideal Torque Source
  w : PMIOPort  Side=Left
  R : PMIOPort  Port=2  Side=Left
  T : PMIOPort  Port=3  Side=Right
  C : PMIOPort  Port=4  Side=Right
  connections:
  T/RConn1 -- Torque Source/RConn1
  w/RConn1 -- Motion Sensor/RConn2
  Motion Sensor/LConn1 -- R/RConn1 -- Torque Source/LConn1
  C/RConn1 -- Torque Source/RConn2 -- Motion Sensor/RConn1

== system AUDI/Eletric motor/PMSM/Voltage Current Interface ==
  Controlled Current Source : fl_lib/Electrical/Electrical Sources/Controlled Current Source
  Voltage Sensor : fl_lib/Electrical/Electrical Sensors/Voltage Sensor
  + : PMIOPort  Side=Left
  - : PMIOPort  Port=2  Side=Right
  i : PMIOPort  Port=3  Side=Right
  V : PMIOPort  Port=4  Side=Left
  connections:
  Voltage Sensor/RConn2 -- Controlled Current Source/LConn1 -- -/RConn1
  i/RConn1 -- Controlled Current Source/RConn1
  Voltage Sensor/RConn1 -- V/RConn1
  +/RConn1 -- Voltage Sensor/LConn1 -- Controlled Current Source/RConn2
